simulink model "fig9_70and71"  (Simulink 4.00)
settings: Solver=ode45  StartTime=0.0  StopTime=20.0  RelTol=1e-5
values from neighbouring files (symbols this model uses):
  f = [0 1 0 0;-k(2)/m(2) -b(2)/m(2) k(2)/m(2) b(2)/m(2) ... (first row only)    [TWOMASS.M]
  g = [0 0 0 1/m(1)]'    [TWOMASS.M]    (also in fig2_12.m = 9.81)
undefined symbols (not defined in the file or in its folder): ac, bc, cc, dc, h2, ht
libraries: simulink3 x1
settings Model: LastModifiedBy=abbas  BlockReductionOpt=off

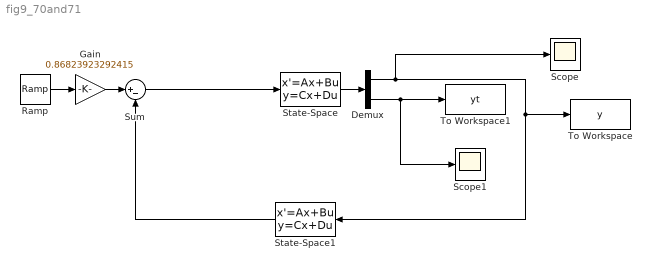
== system fig9_70and71 ==
  Demux : Demux  Outputs=2  BusSelectionMode=off
  Gain : Gain  Gain=0.86823923292415  Multiplication=Element-wise(K.*u)  SaturateOnIntegerOverflow=on
  Ramp : simulink3/Sources/Ramp  slope=1  start=0  X0=0
  Scope : Scope
      settings: TimeRange=auto  YMin=-5  YMax=5  SaveToWorkspace=off  SaveName=ScopeData  LimitDataPoints=on  MaxDataPoints=5000
  Scope1 : Scope
      settings: TimeRange=auto  YMin=-5  YMax=5  SaveToWorkspace=off  LimitDataPoints=on  MaxDataPoints=5000
  State-Space : StateSpace  A=f  B=g  C=[h2;ht]  D=[0;0]  X0=0  Realization=auto  AbsoluteTolerance=auto
  State-Space1 : StateSpace  Orientation=left  A=ac  B=bc  C=cc  D=dc  X0=0  Realization=auto  AbsoluteTolerance=auto
  Sum : Sum  Inputs=|+-  SaturateOnIntegerOverflow=on
  To Workspace : ToWorkspace  VariableName=y  SampleTime=-1  SaveFormat=Array
  To Workspace1 : ToWorkspace  VariableName=yt  SampleTime=-1  SaveFormat=Array
  wires:
  Gain/1 -> Sum/1
  State-Space/1 -> Demux/1
  Demux/1 -> Scope/1, To Workspace/1, State-Space1/1
  Demux/2 -> Scope1/1, To Workspace1/1
  State-Space1/1 -> Sum/2
  Sum/1 -> State-Space/1
  Ramp/1 -> Gain/1
